simulink model "radiator_fan"  (R2023b)
settings: Solver=VariableStepAuto  StartTime=0.0  StopTime=10.0  RelTol=1e-3
settings Model: Creator=Administrator  LastModifiedBy=hp
settings SolverCC: AlgebraicLoopSolver=TrustRegion
settings DebuggingCC: UnconnectedInputMsg=warning  UnconnectedOutputMsg=warning  UnconnectedLineMsg=warning
settings ModelReferenceCC: EnableRefExpFcnMdlSchedulingChecks=on

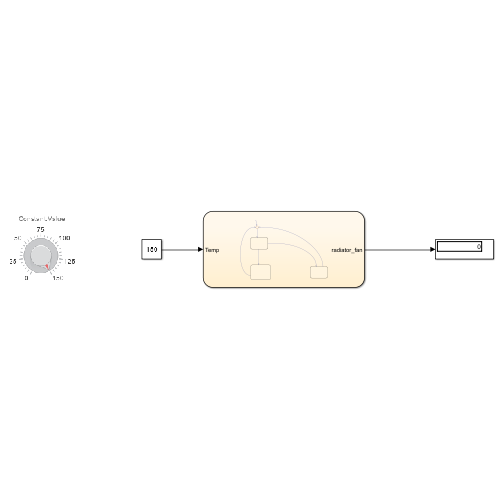
[thumbnail: Simulink's stored preview of the top-level diagram]
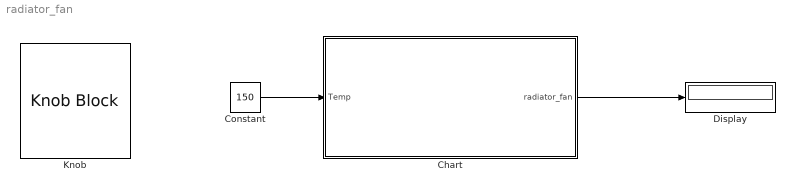
== system radiator_fan ==
  Chart : Stateflow chart  TreatAsAtomicUnit=on
  Constant : Constant  Value=150
  Display : Display
  Knob : KnobBlock  ScaleMax=150
  wires:
  Chart/1(radiator_fan) -> Display/1
  Constant/1 -> Chart/1(Temp)

== stateflow chart radiator_fan/Chart ==
  state Default
    radiator_fan = 0
  state ON_state1
    radiator_fan = 0.5
  state ON_state2
    radiator_fan = 1
  (default) -> (junction 7)
  ON_state1 -> (junction 7) : [Temp<80]
  ON_state2 -> (junction 7) : [Temp<100]
  (junction 7) -> Default
  Default -> ON_state2 [order 2] : [Temp>100]
  Default -> ON_state1 [order 1] : [Temp>80 && Temp<100 ]
  data: Temp input; radiator_fan output
